simulink model "stateSpacewithfilter"  (R2018b)
settings: Solver=ode45  StartTime=0  StopTime=20  MaxStep=1.000000e-02  RelTol=1e-3  EnableMultiTasking=on
undefined symbols (not defined in the file or in its folder): clarinet, flute, oboe
libraries: cstblocks x1
settings Model: Creator=Dan  LastModifiedBy=decla
settings DataIOCC: MaxDataPoints=500  LoadExternalInput=on  SaveFormat=StructureWithTime  SignalLoggingSaveFormat=ModelDataLogs  ReturnWorkspaceOutputs=on
settings OptimizationCC: ExpressionDepthLimit=2147483647  LifeSpan=inf
settings DebuggingCC: AlgebraicLoopMsg=none  UnderspecifiedInitializationDetection=Classic  MergeDetectMultiDrivingBlocksExec=none  FcnCallInpInsideContextMsg=warning  StateNameClashWarn=warning  SFUnexpectedBacktrackingDiag=warning  SFNoUnconditionalDefaultTransitionDiag=warning  SFExecutionAtInitializationDiag=none
settings HardwareCC: ProdBitPerPointer=32  ProdBitPerSizeT=32  ProdBitPerPtrDiffT=32  ProdLargestAtomicFloat=None  ProdIntDivRoundTo=Undefined  ProdEndianess=Unspecified  ProdWordSize=32  ProdHWDeviceType=32-bit Generic
settings ModelReferenceCC: PropagateSignalLabelsOutOfModel=off
settings SFSimCC: SimUseLocalCustomCode=off
settings RTWCC: RTWUseLocalCustomCode=off
settings CodeAppCC: StateflowObjectComments=on
settings GRTTargetCC: TargetLangStandard=C89/C90 (ANSI)  GeneratePreprocessorConditionals=Disable all  CombineOutputUpdateFcns=off  GRTInterface=on
settings ConfigComp: CovMetricSettings=dw  CovHtmlReporting=on  CovSaveCumulativeToWorkspaceVar=on  CovSaveSingleToWorkspaceVar=on  CovExternalEMLEnable=off

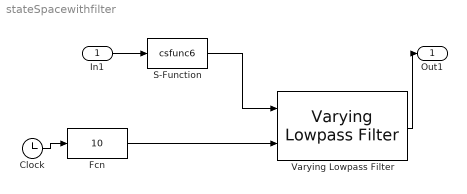
== system stateSpacewithfilter ==
  In1 : Inport
  Clock : Clock
  Fcn : Fcn  Expr=10
  S-Function : S-Function  FunctionName=csfunc6  Parameters=flute,oboe,clarinet  SFunctionDeploymentMode=off  EnableBusSupport=off
  Varying Lowpass Filter : cstblocks/Linear Parameter Varying/Varying Lowpass Filter  N=1
      settings: SourceProductName=Control System Toolbox
  Out1 : Outport
  wires:
  In1/1 -> S-Function/1
  Clock/1 -> Fcn/1
  Fcn/1 -> Varying Lowpass Filter/2
  S-Function/1 -> Varying Lowpass Filter/1
  Varying Lowpass Filter/1 -> Out1/1
